simulink model "SecondKinematic"  (R2023b)
settings: Solver=VariableStepAuto  StartTime=0.0  StopTime=250  RelTol=1e-3
libraries: simulink x2, slpidlib x1
settings Model: Creator=binyh  LastModifiedBy=binyh
settings ModelReferenceCC: ModelReferenceNumInstancesAllowed=Single

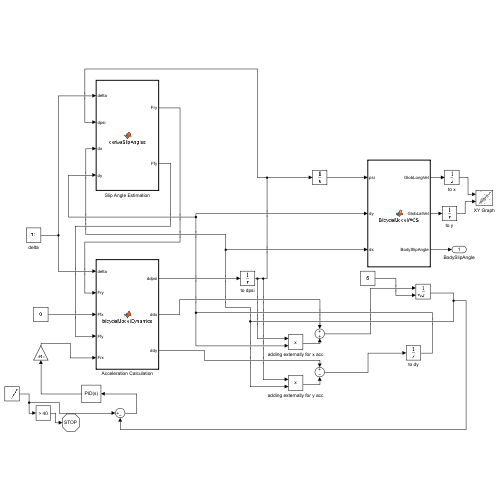
[thumbnail: Simulink's stored preview of the top-level diagram]
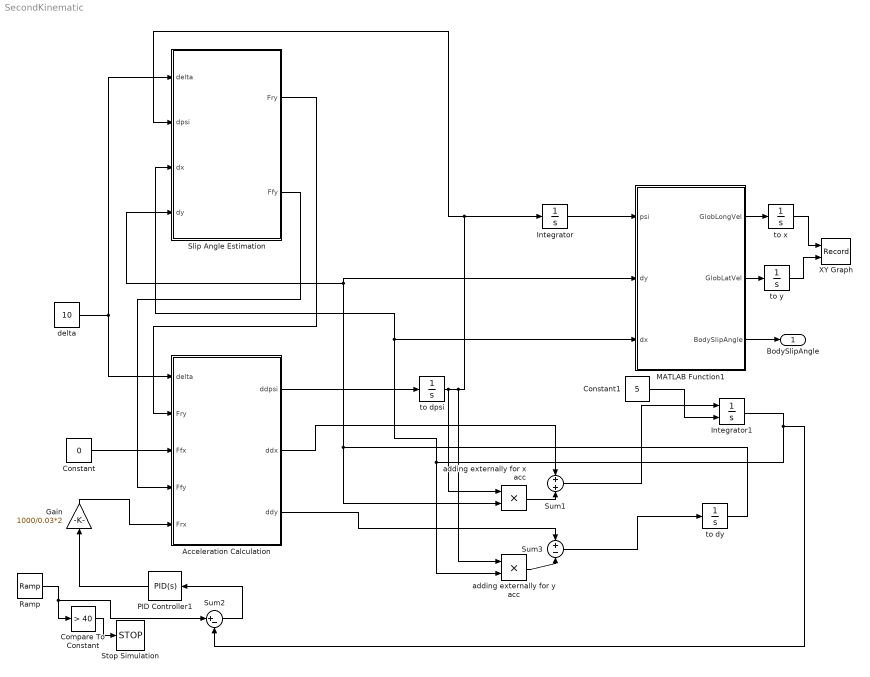
== system SecondKinematic ==
  Acceleration Calculation : MATLAB Function  TreatAsAtomicUnit=on
  Compare To Constant : simulink/Logic and Bit Operations/Compare To Constant  relop=>  const=40  OutDataTypeStr=boolean
  Constant : Constant  Value=0
  Constant1 : Constant  Value=5
  Gain : Gain  Gain=1000/0.03*2
  Integrator : Integrator
  Integrator1 : Integrator  InitialConditionSource=external
  MATLAB Function1 : MATLAB Function  TreatAsAtomicUnit=on
  PID Controller1 : slpidlib/PID Controller  Controller=PID  Form=Parallel  TimeDomain=Continuous-time  UseExternalTs=off  SampleTime=-1  IntegratorMethod=Forward Euler  FilterMethod=Forward Euler  ControllerParametersSource=internal  P=0.0042390143774291  I=0.00081084857567895  UseKiTs=off  D=-0.000893314808680681  N=1.72044274974478  UseFilter=on  TunerSelectOption=Transfer Function Based (PID Tuner App)  InitialConditionSource=internal  InitialConditionForIntegrator=0  InitialConditionForFilter=0  DifferentiatorICPrevScaledInput=0  ExternalReset=none  TrackingMode=off  Kt=1  LimitOutput=off  SatLimitsSource=internal  UpperSaturationLimit=inf  LowerSaturationLimit=-inf  LinearizeAsGain=on  AntiWindupMode=none  Kb=1  LimitIntegrator=off  UpperIntegratorSaturationLimit=inf  LowerIntegratorSaturationLimit=-inf  POutMin=[]  POutMax=[]  IOutMin=[]  IOutMax=[]  DOutMin=[]  DOutMax=[]  NOutMin=[]  NOutMax=[]  SumOutMin=[]  SumOutMax=[]  SaturationOutMin=[]  SaturationOutMax=[]  PParamMin=[]  PParamMax=[]  IParamMin=[]  IParamMax=[]  DParamMin=[]  DParamMax=[]  NParamMin=[]  NParamMax=[]  KbParamMin=[]  KbParamMax=[]  KtParamMin=[]  KtParamMax=[]  KbOutMin=[]  KbOutMax=[]  KtOutMin=[]  KtOutMax=[]  IntegratorOutMin=[]  IntegratorOutMax=[]  FilterOutMin=[]  FilterOutMax=[]  SumI1OutMin=[]  SumI1OutMax=[]  SumI2OutMin=[]  SumI2OutMax=[]  SumI3OutMin=[]  SumI3OutMax=[]  SumI4OutMin=[]  SumI4OutMax=[]  SumDOutMin=[]  SumDOutMax=[]  DifferentiatorOutMin=[]  DifferentiatorOutMax=[]  FilterDiffOutCoefMin=[]  FilterDiffOutCoefMax=[]  ReciprocalOutMin=[]  ReciprocalOutMax=[]  SumDenOutMin=[]  SumDenOutMax=[]  SumNumOutMin=[]  SumNumOutMax=[]  DivideOutMin=[]  DivideOutMax=[]  UdiffTsProdOutMin=[]  UdiffTsProdOutMax=[]  NTsProdOutMin=[]  NTsProdOutMax=[]  UintegralTsProdOutMin=[]  UintegralTsProdOutMax=[]  UngainTsProdOutMin=[]  UngainTsProdOutMax=[]  ClampingZeroOutDataTypeStr=Inherit: Inherit via back propagation  ClampingZeroOutMin=[]  ClampingZeroOutMax=[]  FilterDenConstantOutDataTypeStr=Inherit: Inherit via back propagation  FilterDenConstantOutMin=[]  FilterDenConstantOutMax=[]  PCopyOutDataTypeStr=Inherit: Inherit via back propagation  PCopyOutMin=[]  PCopyOutMax=[]  NCopyOutDataTypeStr=Inherit: Inherit via back propagation  NCopyOutMin=[]  NCopyOutMax=[]  IntegratorContinuousStateAttributes=''  IntegratorStateMustResolveToSignalObject=off  IntegratorRTWStateStorageClass=Auto  FilterContinuousStateAttributes=''  FilterStateMustResolveToSignalObject=off  FilterRTWStateStorageClass=Auto  ParallelPVariant=InternalParameters  IdealPVariant=Disabled  IVariant=InternalParameters  DVariant=InternalParameters  IntegratorVariant=Continuous  SatVariant=Disabled  AWVariant=Passthrough  PCopyVariant=Disabled  TRVariant=Disabled  FdbkBlocksVariant=Forward  IdealPFdbkVariant=Disabled  SatFdbkVariant=Disabled  DerivativeFilterVariant=ContFilter  NVariant=InternalParameters  NCopyVariant=Disabled  FilterICVariant=InternalICsFilter  IntegratorICVariant=InternalICs  ExternalResetVariant=Disabled  TRSumVariant=Passthrough  SumFdbkVariant=Disabled  SumVariant=Sum_PID  TsampFilterVariant=InternalTs  TsampNgainVariant=Passthrough  TsampIntegralVariant=Disabled_SignalSpec  ExternalSaturationOutDataTypeStr=Inherit: Same as second input
  Ramp : simulink/Sources/Ramp  slope=0.05  start=0  InitialOutput=5
  Slip Angle Estimation : MATLAB Function  TreatAsAtomicUnit=on
  Stop Simulation : Stop
  Sum1 : Sum
  Sum2 : Sum  Inputs=|+-
  Sum3 : Sum  Inputs=+-
  XY Graph : Record  FileSettingsInternal="{\"entries\":[{\"content\":{\"excelSettings\":{\"content\":{},\"type\":\"Streamout.ExcelSettings\"}},\"type\":\"Streamout.FileSettingStorage\",\"uuid\":\"\"}],\"packageUris\":[\"http:\\/\\/schema.mathworks.com\\/mf0\\/streamout_blocks\\/R2020a\"],\"version\":\"1.0\"}"  Layout=[1 1]  SignalsInternal="{\"entries\":[{\"content\":{\"signals\":[{\"content\":{\"blockPath\":[],\"dimensions\":[1],\"domain\":\"\",\"lineColor\":\"#a2142f\",\"plots\":[1],\"port\":1,\"sid\":[\"\"],\"signalID\":8899,\"signalName\":\"to x\"},\"type\":\"RecordBlkView.Signal\",\"uuid\":\"\"},{\"content\":{\"blockPath\":[],\"dimensions\":[1],\"domain\":\"\",\"lineColor\":\"#139fff\",\"plots\":[1],\"port\":2,\"sid\":[\"\"],\"signalID\":8903,\"signalName\":\"to y\"},\"type\":\"RecordBlkView.Signal\",\"uuid\":\"\"}]},\"type\":\"RecordBlkView.InputSignals\",\"uuid\":\"\"}],\"packageUris\":[\"http:\\/\\/schema.mathworks.com\\/mf0\\/streamout_blocks\\/R2020a\"],\"version\":\"1.0\"}"  VisualizationBindings="{\"xyplotplugin\":{\"info\":[{\"series\":[{\"bindingParametersList\":[{\"parameter\":\"X-Axis\",\"signalID\":8899,\"signalName\":\"to x\"},{\"parameter\":\"Y-Axis\",\"signalID\":8903,\"signalName\":\"to y\"}],\"seriesID\":13001}],\"subplotID\":1}]}}"  CompatibilityTag=XY
  adding externally for x acc : Product
  adding externally for y acc : Product
  delta : Constant  Value=10
  to dpsi : Integrator
  to dy : Integrator
  to x : Integrator
  to y : Integrator
  BodySlipAngle : Outport
  wires:
  Slip Angle Estimation/1(Fry) -> Acceleration Calculation/2(Fry)
  Slip Angle Estimation/2(Ffy) -> Acceleration Calculation/4(Ffy)
  Acceleration Calculation/1(ddpsi) -> to dpsi/1
  Acceleration Calculation/2(ddx) -> Sum1/1
  Acceleration Calculation/3(ddy) -> Sum3/1
  to dy/1 -> adding externally for x acc/2, MATLAB Function1/2(dy), Slip Angle Estimation/4(dy)
  Integrator1/1 -> Sum2/2, adding externally for y acc/2, Slip Angle Estimation/3(dx), MATLAB Function1/3(dx)
  to dpsi/1 -> Slip Angle Estimation/2(dpsi), Integrator/1, adding externally for y acc/1, adding externally for x acc/1
  delta/1 -> Slip Angle Estimation/1(delta), Acceleration Calculation/1(delta)
  MATLAB Function1/3(BodySlipAngle) -> BodySlipAngle/1
  MATLAB Function1/1(GlobLongVel) -> to x/1
  MATLAB Function1/2(GlobLatVel) -> to y/1
  to y/1 -> XY Graph/2
  to x/1 -> XY Graph/1
  Gain/1 -> Acceleration Calculation/5(Frx)
  Compare To Constant/1 -> Stop Simulation/1
  Ramp/1 -> Sum2/1, Compare To Constant/1
  Constant/1 -> Acceleration Calculation/3(Ffx)
  adding externally for x acc/1 -> Sum1/2
  Sum1/1 -> Integrator1/1
  adding externally for y acc/1 -> Sum3/2
  Sum3/1 -> to dy/1
  Constant1/1 -> Integrator1/2
  Integrator/1 -> MATLAB Function1/1(psi)
  PID Controller1/1 -> Gain/1
  Sum2/1 -> PID Controller1/1

== matlab function SecondKinematic/Slip Angle Estimation ==
  data: delta input; Fry output; dpsi input; dx input; dy input; Ffy output
function [Fry, Ffy] = deriveSlipAngles(delta, dpsi, dx, dy)    
    % Calculating the lateral forces on the front and rear wheels of model 
    % based on the slip angles derived from the vehicle's kinematics. 
    % Takes into account the steering angle (delta), yaw
    % rate, and long and lat velocities.

    % Parameters:
    L = 1.525;          % Total wheelbase: distance from CG to front wheel.
    PercentFront = 0.6; % Percentage distribution of wheelbase at the front.
    k = 400;            % Tire stiffness coefficient.

    % Calculate distances from CG to front and rear wheels.
    Lf = L * (1 - PercentFront); % Distance to the front wheel.
    Lr = L * PercentFront;       % Distance to the rear wheel.

    % Slip angle calculation:
    % angle between the direction of the wheel and direction of travel. 
    % Calculating the front slip angle (alphaF).
    % determined by the steering angle and the difference between the 
    % lateral and longitudinal velocities at the front wheel.
    alphaF = delta - atan2d(dy - (Lf * dpsi), dx);

    % Calculating the rear slip angle (alphaR).
    % Similar to the front, but only influenced by the velocities at the rear wheel.
    alphaR = -atan2d(dy - (Lr * dpsi), dx);
    % Note: The negative sign accounts for the coordinate system used.

    % Calculating the lateral forces based on the slip angles.
    % Tire lateral forces are proportional to the slip angles, with the proportionality
    % constant being the tire stiffness 'k'.
    Fry = k * alphaR; % Lateral force at the rear wheel.
    Ffy = k * alphaF; % Lateral force at the front wheel.
end

== matlab function SecondKinematic/Acceleration Calculation ==
  data: delta input; ddpsi output; Fry input; Ffx input; Ffy input; Frx input; ddx output; ddy output
function [ddpsi, ddx, ddy] = bicycleModelDynamics(delta, Fry, Ffx, Ffy, Frx)
    % Calculating the second derivatives of yaw angle, long. displacement,
    % lat. displacement based on forces and steering angle.

    % Parameters (arbitrary values)
    L = 1.525; % Total wheelbase: distance from center of gravity (CG) to front wheel.
    I = 2.75;   % Vehicle's moment of inertia.
    m = 275;   % Mass of the vehicle in kg.
    PercentFront = 0.6; % Percentage distribution of wheelbase at the front.

    % Dynamics equations
    % Calculating the effective distances to the front (Lf) and rear (Lr) wheels from CG.
    Lf = L * (1 - PercentFront); % Distance from CG to front wheel.
    Lr = L * PercentFront;       % Distance from CG to rear wheel.

    % Calculating the second derivative of yaw angle (ddpsi).
    % It's a measure of how quickly the vehicle is rotating about its vertical axis.
    ddpsi = (-Lr * Fry + Lf * (Ffx * sind(delta) + Ffy * cosd(delta))) / I;

    % Calculating the second derivative of longitudinal displacement (ddx).
    % This is the acceleration in the vehicle's forward direction.
    ddx = (Frx + Ffx * cosd(delta) - Ffy * sind(delta)) / m;

    % Calculating the second derivative of lateral displacement (ddy).
    % This is the acceleration perpendicular to the vehicle's forward direction.
    ddy = (Fry + Ffx * sind(delta) + Ffy * cosd(delta)) / m;
    
end

== matlab function SecondKinematic/MATLAB Function1 ==
  data: psi input; GlobLongVel output; dy input; dx input; GlobLatVel output; BodySlipAngle output
function [GlobLongVel, GlobLatVel, BodySlipAngle] = ...
    BicycleModelWCS( psi, dy, dx )

% Changing coordinates for global velocity
GlobLongVel = dx .* cosd( psi ) - dy .* sind( psi );
GlobLatVel = dx .* sind( psi ) + dy .* cosd( psi );  
                 

% Body Slip
BodySlipAngle = atan2d( dy, dx );

end
